simulink model "svpwm_sfunction_common"  (R2019a)
settings: Solver=ode23tb  StartTime=0.0  StopTime=0.05  MaxStep=0.00001  RelTol=1e-3  EnableMultiTasking=on
InitFcn:
  | Vdc = 100;
libraries: simulink x1
settings Model: Creator=YUAN  LastModifiedBy=Administrator
settings DataIOCC: LimitDataPoints=on  SaveFormat=Array  SignalLoggingSaveFormat=ModelDataLogs  ReturnWorkspaceOutputs=off
settings OptimizationCC: ExpressionDepthLimit=2147483647  LifeSpan=inf
settings DebuggingCC: UnderspecifiedInitializationDetection=Classic  MergeDetectMultiDrivingBlocksExec=none  SolverPrmCheckMsg=warning  FcnCallInpInsideContextMsg=warning  StateNameClashWarn=warning  SFUnexpectedBacktrackingDiag=warning  SFNoUnconditionalDefaultTransitionDiag=warning  SFExecutionAtInitializationDiag=none  ArithmeticOperatorsInVariantConditions=warning
settings HardwareCC: ProdBitPerPointer=32  ProdBitPerSizeT=32  ProdBitPerPtrDiffT=32  ProdLargestAtomicFloat=None  ProdIntDivRoundTo=Undefined  ProdEndianess=Unspecified  ProdWordSize=32  ProdHWDeviceType=32-bit Generic
settings ModelReferenceCC: PropagateSignalLabelsOutOfModel=off
settings SFSimCC: SimUseLocalCustomCode=off
settings RTWCC: RTWUseLocalCustomCode=off
settings CodeAppCC: StateflowObjectComments=on
settings GRTTargetCC: TargetLangStandard=C89/C90 (ANSI)  GeneratePreprocessorConditionals=Disable all  CombineOutputUpdateFcns=off  GRTInterface=on
settings ConfigComp: CovMetricSettings=dw  CovHtmlReporting=on  CovSaveCumulativeToWorkspaceVar=on  CovSaveSingleToWorkspaceVar=on  CovExternalEMLEnable=off

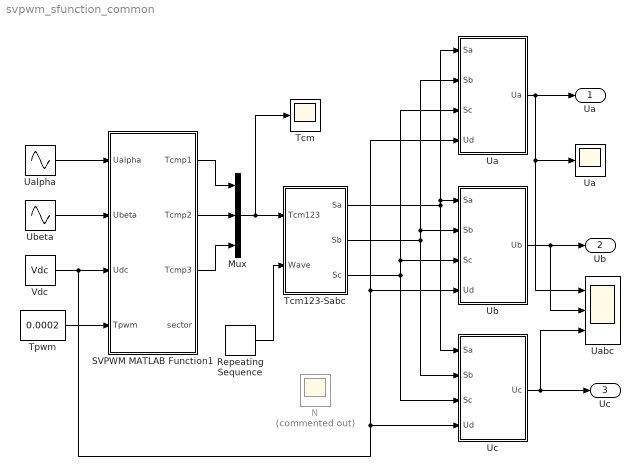
== system svpwm_sfunction_common ==
  Mux : Mux  Inputs=3
  N : Scope  Commented=on
  Repeating Sequence : simulink/Sources/Repeating Sequence  rep_seq_t=[0 1/10000 1/5000]  rep_seq_y=[0 1/10000 0]
  SVPWM MATLAB Function1 : MATLAB Function  TreatAsAtomicUnit=on
  Tcm : Scope
  Tcm123-Sabc : Subsystem
  Tpwm : Constant  Value=0.0002
  "Ua " : Subsystem
  "Ua  " : Scope
  Uabc : Scope  NumInputPorts=3
  Ualpha : Sin  Amplitude=Vdc/sqrt(3)  Frequency=100*pi  Phase=pi/2
  "Ub " : Subsystem
  Ubeta : Sin  Amplitude=Vdc/sqrt(3)  Frequency=100*pi
  "Uc  " : Subsystem
  Vdc : Constant  Value=Vdc
  Ua : Outport
  Ub : Outport  Port=2
  Uc : Outport  Port=3
  wires:
  Ualpha/1 -> SVPWM MATLAB Function1/1(Ualpha)
  Ubeta/1 -> SVPWM MATLAB Function1/2(Ubeta)
  Tpwm/1 -> SVPWM MATLAB Function1/4(Tpwm)
  Mux/1 -> Tcm123-Sabc/1(Tcm123), Tcm/1
  Repeating Sequence/1 -> Tcm123-Sabc/2(Wave)
  Tcm123-Sabc/1(Sa) -> "Ua "/1(Sa), "Ub "/1(Sa), "Uc  "/1("Sa ")
  Tcm123-Sabc/2(Sb) -> "Ua "/2(Sb), "Ub "/2(Sb), "Uc  "/2(Sb)
  Tcm123-Sabc/3(Sc) -> "Ua "/3(Sc), "Ub "/3(Sc), "Uc  "/3(Sc)
  "Ua "/1(Ua) -> Uabc/1, "Ua  "/1, Ua/1
  "Ub "/1(Ub) -> Uabc/2, Ub/1
  "Uc  "/1(Uc) -> Uc/1, Uabc/3
  Vdc/1 -> SVPWM MATLAB Function1/3(Udc), "Uc  "/4(Ud), "Ua "/4(Ud), "Ub "/4(Ud)
  SVPWM MATLAB Function1/2(Tcmp2) -> Mux/2
  SVPWM MATLAB Function1/3(Tcmp3) -> Mux/3
  SVPWM MATLAB Function1/1(Tcmp1) -> Mux/1

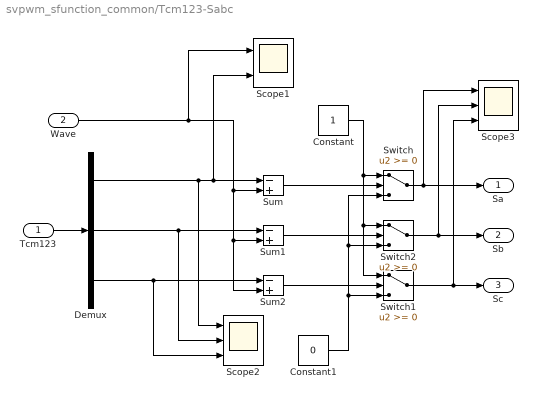
== system svpwm_sfunction_common/Tcm123-Sabc ==
  Tcm123 : Inport
  Wave : Inport  Port=2
  Constant : Constant
  Constant1 : Constant  Value=0
  Demux : Demux  Outputs=3
  Scope1 : Scope  NumInputPorts=2
  Scope2 : Scope  NumInputPorts=3
  Scope3 : Scope  NumInputPorts=3
  Sum : Sum  Inputs=-+  SaturateOnIntegerOverflow=on
  Sum1 : Sum  Inputs=-+  SaturateOnIntegerOverflow=on
  Sum2 : Sum  Inputs=-+  SaturateOnIntegerOverflow=on
  Switch : Switch  SaturateOnIntegerOverflow=on
  Switch1 : Switch  SaturateOnIntegerOverflow=on
  Switch2 : Switch  SaturateOnIntegerOverflow=on
  Sa : Outport
  Sb : Outport  Port=2
  Sc : Outport  Port=3
  wires:
  Switch1/1 -> Sc/1, Scope3/3
  Switch2/1 -> Sb/1, Scope3/2
  Switch/1 -> Sa/1, Scope3/1
  Constant1/1 -> Switch1/3, Switch2/3, Switch/3
  Constant/1 -> Switch/1, Switch2/1, Switch1/1
  Sum2/1 -> Switch1/2
  Sum1/1 -> Switch2/2
  Sum/1 -> Switch/2
  Tcm123/1 -> Demux/1
  Demux/3 -> Sum2/1, Scope2/3
  Demux/2 -> Sum1/1, Scope2/2
  Demux/1 -> Scope1/2, Sum/1, Scope2/1
  Wave/1 -> Sum1/2, Sum2/2, Sum/2, Scope1/1

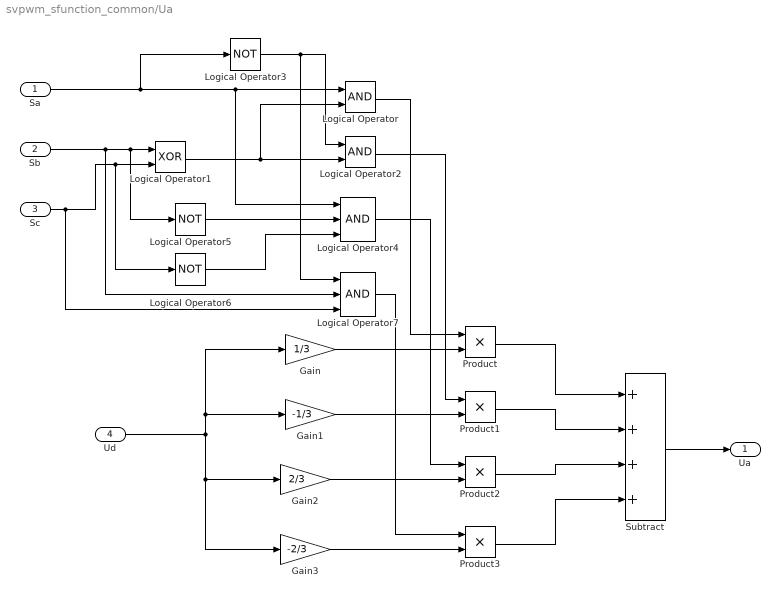
== system svpwm_sfunction_common/Ua  ==
  Sa : Inport
  Sb : Inport  Port=2
  Sc : Inport  Port=3
  Ud : Inport  Port=4
  Gain : Gain  Gain=1/3
  Gain1 : Gain  Gain=-1/3
  Gain2 : Gain  Gain=2/3
  Gain3 : Gain  Gain=-2/3
  Logical Operator : Logic  AllPortsSameDT=off  OutDataTypeStr=boolean
  Logical Operator1 : Logic  Operator=XOR  AllPortsSameDT=off  OutDataTypeStr=boolean
  Logical Operator2 : Logic  AllPortsSameDT=off  OutDataTypeStr=boolean
  Logical Operator3 : Logic  Operator=NOT  AllPortsSameDT=off  OutDataTypeStr=boolean
  Logical Operator4 : Logic  Inputs=3  AllPortsSameDT=off  OutDataTypeStr=boolean
  Logical Operator5 : Logic  Operator=NOT  AllPortsSameDT=off  OutDataTypeStr=boolean
  Logical Operator6 : Logic  Operator=NOT  AllPortsSameDT=off  OutDataTypeStr=boolean
  Logical Operator7 : Logic  Inputs=3  AllPortsSameDT=off  OutDataTypeStr=boolean
  Product{,1..3} (4 alike) : Product  RndMeth=Zero
  Subtract : Sum  Inputs=++++
  Ua : Outport
  wires:
  Ud/1 -> Gain3/1, Gain2/1, Gain1/1, Gain/1
  Gain/1 -> Product/2
  Gain1/1 -> Product1/2
  Gain2/1 -> Product2/2
  Gain3/1 -> Product3/2
  Product/1 -> Subtract/1
  Product1/1 -> Subtract/2
  Product2/1 -> Subtract/3
  Product3/1 -> Subtract/4
  Subtract/1 -> Ua/1
  Logical Operator/1 -> Product/1
  Sa/1 -> Logical Operator4/1, Logical Operator/1, Logical Operator3/1
  Sb/1 -> Logical Operator7/2, Logical Operator5/1, Logical Operator1/1
  Sc/1 -> Logical Operator7/3, Logical Operator6/1, Logical Operator1/2
  Logical Operator1/1 -> Logical Operator/2, Logical Operator2/2
  Logical Operator2/1 -> Product1/1
  Logical Operator3/1 -> Logical Operator2/1, Logical Operator7/1
  Logical Operator4/1 -> Product2/1
  Logical Operator5/1 -> Logical Operator4/2
  Logical Operator6/1 -> Logical Operator4/3
  Logical Operator7/1 -> Product3/1

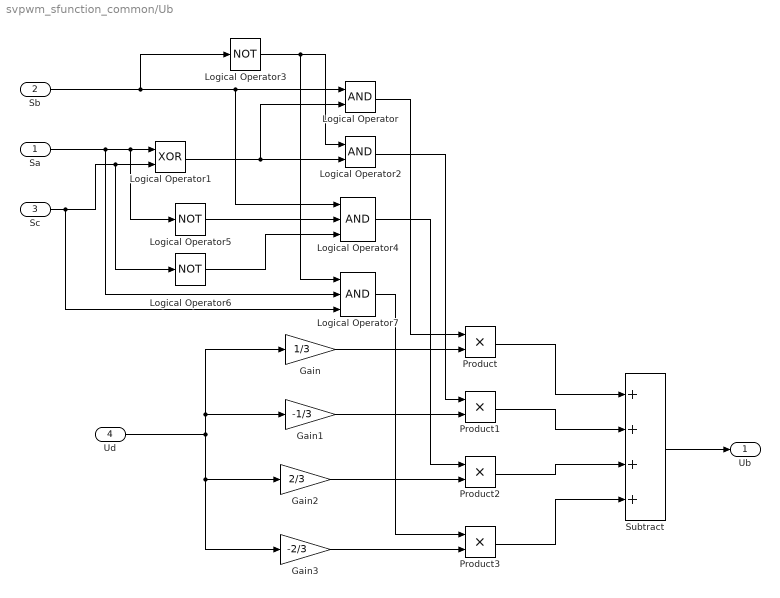
== system svpwm_sfunction_common/Ub  ==
  Sa : Inport
  Sb : Inport  Port=2
  Sc : Inport  Port=3
  Ud : Inport  Port=4
  Gain : Gain  Gain=1/3
  Gain1 : Gain  Gain=-1/3
  Gain2 : Gain  Gain=2/3
  Gain3 : Gain  Gain=-2/3
  Logical Operator : Logic  AllPortsSameDT=off  OutDataTypeStr=boolean
  Logical Operator1 : Logic  Operator=XOR  AllPortsSameDT=off  OutDataTypeStr=boolean
  Logical Operator2 : Logic  AllPortsSameDT=off  OutDataTypeStr=boolean
  Logical Operator3 : Logic  Operator=NOT  AllPortsSameDT=off  OutDataTypeStr=boolean
  Logical Operator4 : Logic  Inputs=3  AllPortsSameDT=off  OutDataTypeStr=boolean
  Logical Operator5 : Logic  Operator=NOT  AllPortsSameDT=off  OutDataTypeStr=boolean
  Logical Operator6 : Logic  Operator=NOT  AllPortsSameDT=off  OutDataTypeStr=boolean
  Logical Operator7 : Logic  Inputs=3  AllPortsSameDT=off  OutDataTypeStr=boolean
  Product{,1..3} (4 alike) : Product  RndMeth=Zero
  Subtract : Sum  Inputs=++++
  Ub : Outport
  wires:
  Ud/1 -> Gain3/1, Gain2/1, Gain1/1, Gain/1
  Gain/1 -> Product/2
  Gain1/1 -> Product1/2
  Gain2/1 -> Product2/2
  Gain3/1 -> Product3/2
  Product/1 -> Subtract/1
  Product1/1 -> Subtract/2
  Product2/1 -> Subtract/3
  Product3/1 -> Subtract/4
  Subtract/1 -> Ub/1
  Logical Operator/1 -> Product/1
  Sb/1 -> Logical Operator4/1, Logical Operator/1, Logical Operator3/1
  Sa/1 -> Logical Operator7/2, Logical Operator5/1, Logical Operator1/1
  Sc/1 -> Logical Operator7/3, Logical Operator6/1, Logical Operator1/2
  Logical Operator1/1 -> Logical Operator/2, Logical Operator2/2
  Logical Operator2/1 -> Product1/1
  Logical Operator3/1 -> Logical Operator2/1, Logical Operator7/1
  Logical Operator4/1 -> Product2/1
  Logical Operator5/1 -> Logical Operator4/2
  Logical Operator6/1 -> Logical Operator4/3
  Logical Operator7/1 -> Product3/1

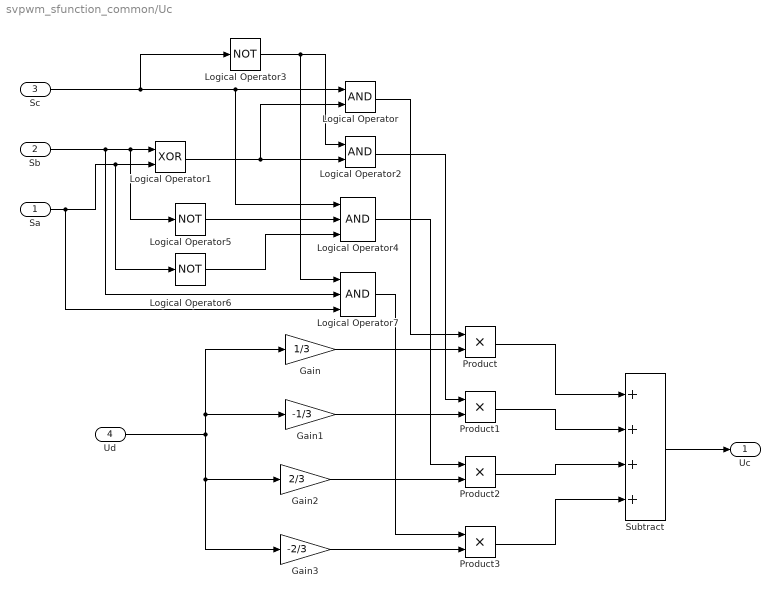
== system svpwm_sfunction_common/Uc   ==
  "Sa " : Inport
  Sb : Inport  Port=2
  Sc : Inport  Port=3
  Ud : Inport  Port=4
  Gain : Gain  Gain=1/3
  Gain1 : Gain  Gain=-1/3
  Gain2 : Gain  Gain=2/3
  Gain3 : Gain  Gain=-2/3
  Logical Operator : Logic  AllPortsSameDT=off  OutDataTypeStr=boolean
  Logical Operator1 : Logic  Operator=XOR  AllPortsSameDT=off  OutDataTypeStr=boolean
  Logical Operator2 : Logic  AllPortsSameDT=off  OutDataTypeStr=boolean
  Logical Operator3 : Logic  Operator=NOT  AllPortsSameDT=off  OutDataTypeStr=boolean
  Logical Operator4 : Logic  Inputs=3  AllPortsSameDT=off  OutDataTypeStr=boolean
  Logical Operator5 : Logic  Operator=NOT  AllPortsSameDT=off  OutDataTypeStr=boolean
  Logical Operator6 : Logic  Operator=NOT  AllPortsSameDT=off  OutDataTypeStr=boolean
  Logical Operator7 : Logic  Inputs=3  AllPortsSameDT=off  OutDataTypeStr=boolean
  Product{,1..3} (4 alike) : Product  RndMeth=Zero
  Subtract : Sum  Inputs=++++
  Uc : Outport
  wires:
  Ud/1 -> Gain3/1, Gain2/1, Gain1/1, Gain/1
  Gain/1 -> Product/2
  Gain1/1 -> Product1/2
  Gain2/1 -> Product2/2
  Gain3/1 -> Product3/2
  Product/1 -> Subtract/1
  Product1/1 -> Subtract/2
  Product2/1 -> Subtract/3
  Product3/1 -> Subtract/4
  Subtract/1 -> Uc/1
  Logical Operator/1 -> Product/1
  Sc/1 -> Logical Operator4/1, Logical Operator/1, Logical Operator3/1
  Sb/1 -> Logical Operator7/2, Logical Operator5/1, Logical Operator1/1
  "Sa "/1 -> Logical Operator7/3, Logical Operator6/1, Logical Operator1/2
  Logical Operator1/1 -> Logical Operator/2, Logical Operator2/2
  Logical Operator2/1 -> Product1/1
  Logical Operator3/1 -> Logical Operator2/1, Logical Operator7/1
  Logical Operator4/1 -> Product2/1
  Logical Operator5/1 -> Logical Operator4/2
  Logical Operator6/1 -> Logical Operator4/3
  Logical Operator7/1 -> Product3/1

== matlab function svpwm_sfunction_common/SVPWM MATLAB Function1 ==
  data: Ualpha input; Tcmp1 output; Ubeta input; Tcmp2 output; Tcmp3 output; Udc input; Tpwm input; sector output
function [Tcmp1,Tcmp2,Tcmp3,sector] = fcn(Ualpha,Ubeta,Udc,Tpwm)
%#codegen
SVGEN_SQRT3_OVER_2 = (0.8660254038);
SVGEN_SQRT3  = 1.7321;
UmodBase = Udc/2;
% UmodBase = Udc;
% UmodBase = 1;

Va_tmp = -(Ualpha*(0.5))/UmodBase;
Vb_tmp = (SVGEN_SQRT3_OVER_2*Ubeta)/UmodBase;

Va = Ualpha/UmodBase;  %alpha
Vb = Va_tmp + Vb_tmp; %-0.5*alpha + sqrt(3)/2 * beta;
Vc = Va_tmp - Vb_tmp; %-0.5*alpha - sqrt(3)/2 * beta;

% find order Vmin,Vmid,Vmax
if (Va > Vb)
Vmax = Va;
Vmin = Vb;
else
Vmax = Vb;
Vmin = Va;
end

if Vc > Vmax
Vmax = Vc;
elseif (Vc < Vmin)
Vmin = Vc;
end

Vcom = ((Vmax+Vmin)*(0.5));

% Subtract common-mode term to achieve SV modulation
Ta = (Va - Vcom);
Tb = (Vb - Vcom);
Tc = (Vc - Vcom); 
  
% Ta = Ta/SVGEN_SQRT3_OVER_2 ;
% Tb = Tb/SVGEN_SQRT3_OVER_2 ;
% Tc = Tc/SVGEN_SQRT3_OVER_2 ;
% %(-1,1) to (0,1),similar to Mfuncx
Ta = Ta/2 + 0.5;
Tb = Tb/2 + 0.5;
Tc = Tc/2 + 0.5;

%dutycycle :(-0.5,0.5) to (0,1)
% Ta = Ta + 0.5;
% Tb = Tb + 0.5;
% Tc = Tc + 0.5;
%duty to switch instant
Tcmp1 = (1 - Ta)*Tpwm/2;
Tcmp2 = (1 - Tb)*Tpwm/2;
Tcmp3 = (1 - Tc)*Tpwm/2;

sector = 0;
end
